simulink model "dc_motor_model"  (R2023a)
settings: Solver=VariableStepAuto  StartTime=0.0  StopTime=5  RelTol=1e-3
undefined symbols (not defined in the file): B, J, Kb, Ki, Kp, Kt, L, R
settings Model: Creator=Acer  LastModifiedBy=Acer

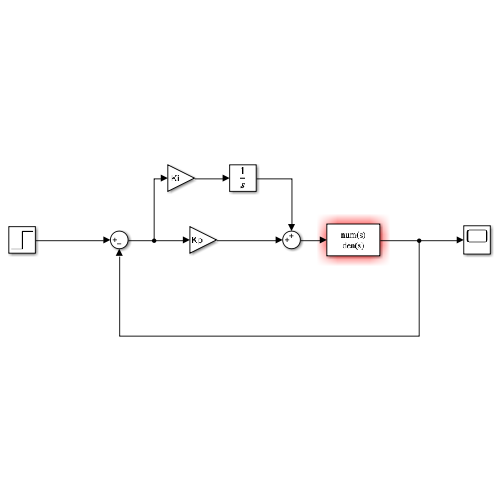
[thumbnail: Simulink's stored preview of the top-level diagram]
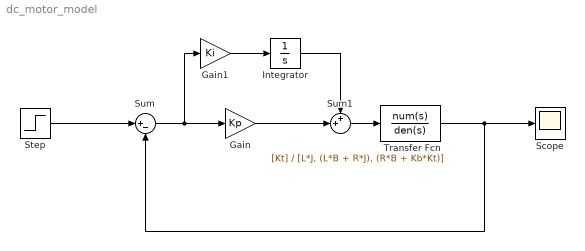
== system dc_motor_model ==
  Gain : Gain  Gain=Kp
  Gain1 : Gain  Gain=Ki
  Integrator : Integrator
  Scope : Scope
  Step : Step  Before=1  SampleTime=0
  Sum : Sum  Inputs=|+-
  Sum1 : Sum  Inputs=++|
  Transfer Fcn : TransferFcn  Numerator=[Kt]  Denominator=[L*J, (L*B + R*J), (R*B + Kb*Kt)]
  wires:
  Transfer Fcn/1 -> Sum/2, Scope/1
  Step/1 -> Sum/1
  Sum/1 -> Gain/1, Gain1/1
  Sum1/1 -> Transfer Fcn/1
  Integrator/1 -> Sum1/1
  Gain/1 -> Sum1/2
  Gain1/1 -> Integrator/1
